simulink model "motor_cardynamic"  (R2020b)
settings: Solver=VariableStepAuto  StartTime=0.0  StopTime=10.0  RelTol=1e-3
values from neighbouring files (symbols this model uses):
  A = 2.34/64    (= 0.0365625)    [car_model_parameters.m]
  Cd = 0.3    [car_model_parameters.m]
  g = 9.81    [car_model_parameters.m]
  Gr = 2.5    [car_model_parameters.m]
  Ke = 0.023    [car_model_parameters.m]
  Kt = 0.023    [car_model_parameters.m]
  L = 0.5    [car_model_parameters.m]
  m = 1.5    [car_model_parameters.m]
  R = 1    [car_model_parameters.m]
  r = 3.2*1e-2    (= 0.032)    [car_model_parameters.m]
  rho = 1.204    [car_model_parameters.m]
settings Model: Creator=arthur  LastModifiedBy=arthur

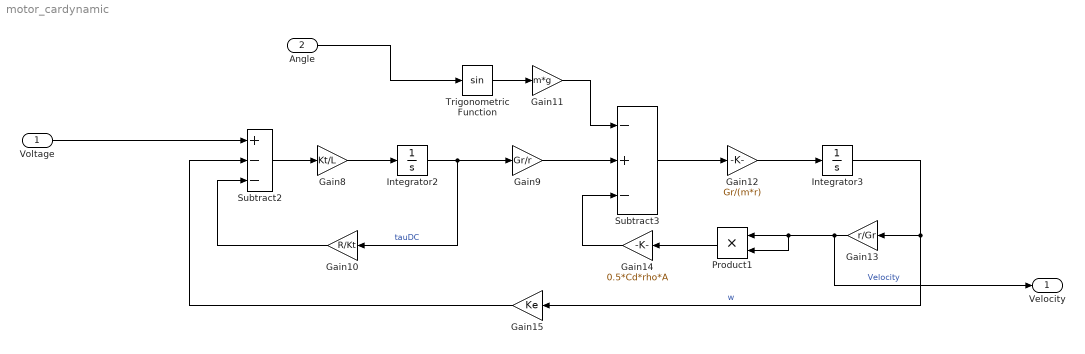
== system motor_cardynamic ==
  Voltage : Inport
  Angle : Inport  Port=2
  Gain10 : Gain  Gain=R/Kt
  Gain11 : Gain  Gain=m*g
  Gain12 : Gain  Gain=Gr/(m*r)
  Gain13 : Gain  Gain=r/Gr
  Gain14 : Gain  Gain=0.5*Cd*rho*A
  Gain15 : Gain  Gain=Ke
  Gain8 : Gain  Gain=Kt/L
  Gain9 : Gain  Gain=Gr/r
  Integrator2 : Integrator
  Integrator3 : Integrator
  Product1 : Product
  Subtract2 : Sum  Inputs=+--
  Subtract3 : Sum  Inputs=-+-
  Trigonometric Function : Trigonometry
  Velocity : Outport
  wires:
  Subtract2/1 -> Gain8/1
  Gain8/1 -> Integrator2/1
  Integrator2/1 -> Gain9/1, Gain10/1  "tauDC"
  Gain10/1 -> Subtract2/3
  Trigonometric Function/1 -> Gain11/1
  Subtract3/1 -> Gain12/1
  Gain12/1 -> Integrator3/1
  Integrator3/1 -> Gain15/1, Gain13/1  "w"
  Gain13/1 -> Velocity/1, Product1/1, Product1/2  "Velocity"
  Product1/1 -> Gain14/1
  Gain14/1 -> Subtract3/3
  Gain15/1 -> Subtract2/2
  Gain9/1 -> Subtract3/2
  Angle/1 -> Trigonometric Function/1
  Voltage/1 -> Subtract2/1
  Gain11/1 -> Subtract3/1
